simulink model "dsbsc"  (Simulink 5.0)
settings: Solver=ode45  StartTime=0.0  StopTime=7  RelTol=1e-3
libraries: dsparch4 x2, dspsigops x2, dspwin32 x2, commnoisgen2 x1
settings Model: LastModifiedBy=Daiming Qu

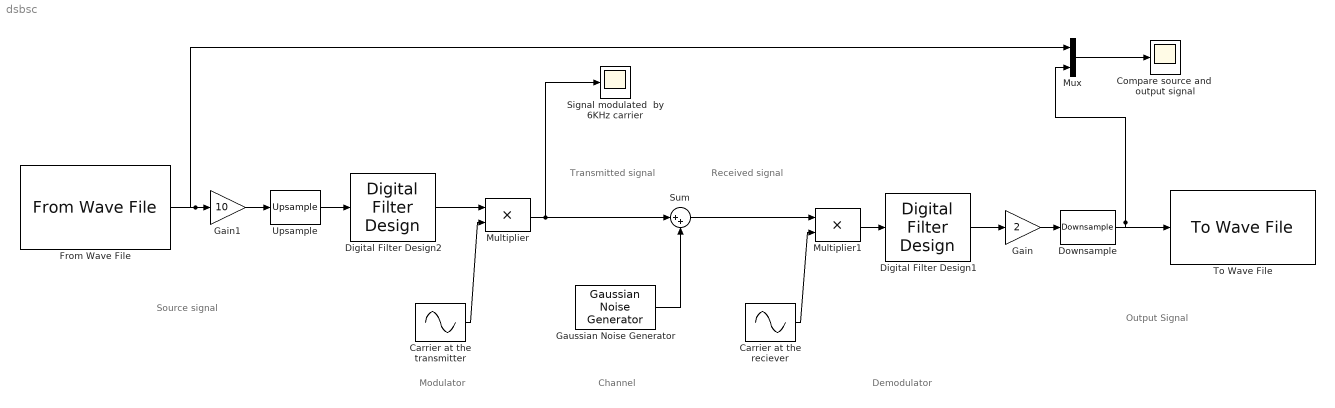
== system dsbsc ==
  note: Source signal
  note: Output Signal
  note: Transmitted
      | signal
  note: Modulator
  note: Demodulator
  note: Received
      | signal
  note: Channel
  Carrier at the reciever : Sin  Frequency=2*pi*6000  Phase=pi/2  SampleTime=1/240000
  Carrier at the transmitter : Sin  Frequency=2*pi*6000  Phase=pi/2  SampleTime=1/240000
  Compare source and  output signal : Scope
      settings: YMin=-0.000425  YMax=0.000125  SaveName=ScopeData3  MaxDataPoints=50000
  Digital Filter Design1 : dsparch4/Digital Filter Design
  Digital Filter Design2 : dsparch4/Digital Filter Design
  Downsample : dspsigops/Downsample  N=10  phase=0  ic=0  smode=Allow multirate  fmode=Maintain input frame size
  From Wave File : dspwin32/From Wave File  FileName=speech_dian.wav  SamplesPerFrame=1  MinBufSize=256  dType=Double
  Gain : Gain  Gain=2  SaturateOnIntegerOverflow=on
  Gain1 : Gain  Gain=10  SaturateOnIntegerOverflow=on
  Gaussian Noise Generator : commnoisgen2/Gaussian Noise Generator  m=0  d=0.0000001  s=41  Ts=1/240000  frameBased=off  sampPerFrame=1  orient=off
  Multiplier : Product  SaturateOnIntegerOverflow=on
  Multiplier1 : Product  SaturateOnIntegerOverflow=on
  Mux : Mux  Inputs=2
  Signal modulated  by 6KHz carrier : Scope
  Sum : Sum  Inputs=|++  SaturateOnIntegerOverflow=on
  To Wave File : dspwin32/To Wave File  filename=speech_rcv  sampleWidth=16  MinNumSamples=256
  Upsample : dspsigops/Upsample  N=10  phase=0  ic=0  mode=Maintain input frame size
  wires:
  Carrier at the transmitter/1 -> Multiplier/2
  Carrier at the reciever/1 -> Multiplier1/2
  Mux/1 -> Compare source and  output signal/1
  Gain/1 -> Downsample/1
  From Wave File/1 -> Mux/1, Gain1/1
  Multiplier1/1 -> Digital Filter Design1/1
  Multiplier/1 -> Signal modulated  by 6KHz carrier/1, Sum/1
  Digital Filter Design1/1 -> Gain/1
  Digital Filter Design2/1 -> Multiplier/1
  Upsample/1 -> Digital Filter Design2/1
  Downsample/1 -> Mux/2, To Wave File/1
  Sum/1 -> Multiplier1/1
  Gaussian Noise Generator/1 -> Sum/2
  Gain1/1 -> Upsample/1
